simulink model "sim_part1"  (R2021a)
settings: Solver=VariableStepAuto  StartTime=0.0  StopTime=10  RelTol=1e-3
values from neighbouring files (symbols this model uses):
  A = [0 1 0 0; 0 0 -m*g / M 0; 0 0 0 1; 0 0 (M+m)*g/(M*l) 0]    [prelab.m]
  B = [0; 1/M; 0; -1/(M*l)]    [prelab.m]
  C = eye(4)    [prelab.m]
  D = [0;0;0;0]    [prelab.m]
libraries: truetime x1
settings Model: Creator=lixinru  LastModifiedBy=lixinru

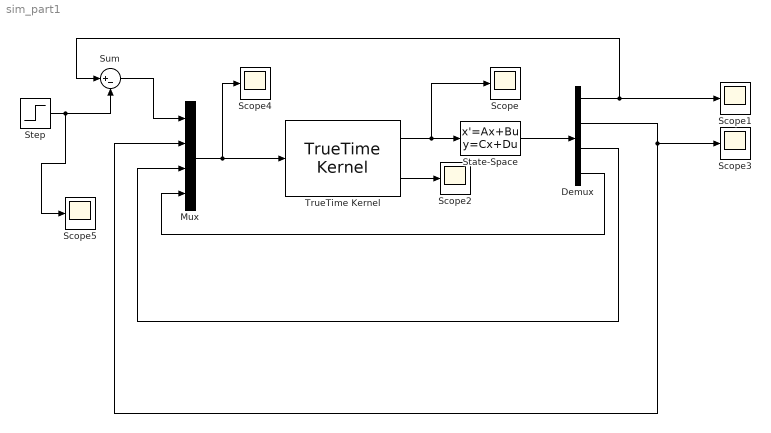
== system sim_part1 ==
  Demux : Demux
  Mux : Mux
  Scope{,1..5} (6 alike) : Scope
  State-Space : StateSpace  A=A  B=B  C=C  D=D  InitialCondition=0
  Step : Step  Time=0  Before=1  SampleTime=0
  Sum : Sum  Inputs=|+-
  TrueTime Kernel : truetime/TrueTime Kernel  sfun=simple_init  args=[]  ninputsoutputs=[4 1]  ntriggers=0  trigtype=falling  nwnodenbr=[]  clockoffsetdrift=[0 0]  schedoutput=on  battery=off  poweroutput=off
  wires:
  State-Space/1 -> Demux/1
  Demux/1 -> Sum/1, Scope1/1
  Demux/4 -> Mux/4
  Demux/3 -> Mux/3
  Demux/2 -> Scope3/1, Mux/2
  Sum/1 -> Mux/1
  Step/1 -> Scope5/1, Sum/2
  Mux/1 -> TrueTime Kernel/1, Scope4/1
  TrueTime Kernel/1 -> Scope/1, State-Space/1
  TrueTime Kernel/2 -> Scope2/1
